simulink model "Phase2_Model"  (R2022b)
settings: Solver=ode4  StartTime=0.0  StopTime=40  FixedStep=Ts  RelTol=1e-3
values from neighbouring files (symbols this model uses):
  b1 = 0.001    [param.m]
  b2 = 1e-5    (= 1e-05)    [param.m]
  g = 9.81    [param.m]
  J1 = (1/12)*m1*L1^2    (= 7.91666666667e-05)    [param.m]
  J2 = (1/12)*m2*L2^2    (= 3.3282e-05)    [param.m]
  km = 0.042    [param.m]
  L1 = 0.1    [param.m]
  l1 = L1/2    (= 0.05)    [param.m]
  L2 = 0.129    [param.m]
  l2 = L2/2    (= 0.0645)    [param.m]
  m1 = 0.095    [param.m]
  m2 = 0.024    [param.m]
  Rm = 8.4    [param.m]
  X0 = [q10; q20-pi/10; q1dot0; q2dot0]    [param.m]
undefined symbols (not defined in the file or in its folder): k, sum_amps, sum_freqs, sum_gains
settings Model: Creator=shahin  LastModifiedBy=ranir
settings DataIOCC: ReturnWorkspaceOutputs=off

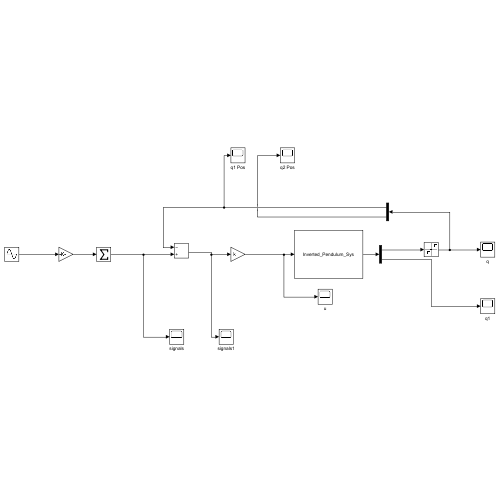
[thumbnail: Simulink's stored preview of the top-level diagram]
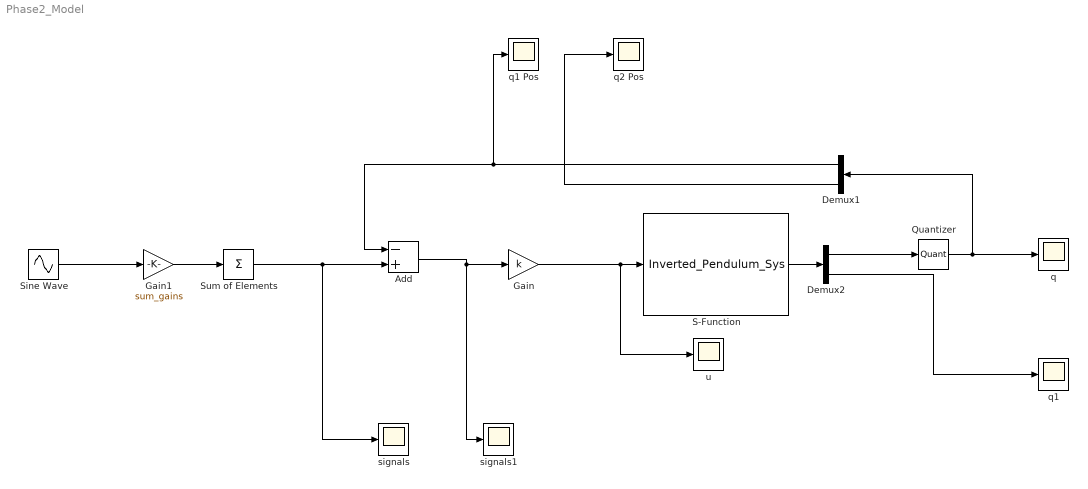
== system Phase2_Model ==
  Add : Sum  Inputs=-+
  Demux1 : Demux  Outputs=2
  Demux2 : Demux  Outputs=2
  Gain : Gain  Gain=k
  Gain1 : Gain  Gain=sum_gains
  Quantizer : Quantizer  QuantizationInterval="[2*pi/2048  2*pi/2048]"
  S-Function : S-Function  FunctionName=Inverted_Pendulum_Sys  Parameters=X0,L1,L2,l1,l2,m1,m2,J1,J2,g,b1,b2,km,Rm  SFunctionDeploymentMode=off  EnableBusSupport=off
  Sine Wave : Sin  Amplitude=sum_amps  Frequency=sum_freqs  SampleTime=0
  Sum of Elements : Sum  Inputs=+
  q : Scope
  q1 : Scope
  q1 Pos : Scope
  q2 Pos : Scope
  signals : Scope
  signals1 : Scope
  u : Scope
  wires:
  Demux2/1 -> Quantizer/1
  S-Function/1 -> Demux2/1
  Quantizer/1 -> q/1, Demux1/1
  Demux1/1 -> Add/1, q1 Pos/1
  Add/1 -> signals1/1, Gain/1
  Demux1/2 -> q2 Pos/1
  Demux2/2 -> q1/1
  Gain/1 -> u/1, S-Function/1
  Gain1/1 -> Sum of Elements/1
  Sine Wave/1 -> Gain1/1
  Sum of Elements/1 -> signals/1, Add/2
